simulink model "SAC_est_2d_test"  (R2025b)
settings: Solver=VariableStepAuto  StartTime=0.0  StopTime=300  FixedStep=1e-4  RelTol=1e-5
InitFcn:
  | % InitFcn (Model Properties > Callbacks > InitFcn)
  | 
  | % モデルファイルのフルパス（未保存だと空になるので注意）
  | % そのフォルダをパスに追加（重複追加はMATLAB側である程度防がれますが念のため）
  | modelDir = fileparts(get_param(bdroot, 'FileName'));
  | if ~contains(path, modelDir)
  |     addpath(modelDir);
  | end
  | 
  | % 呼びたい関数（そのフォルダ内に my_init.m がある想定）
  | model_init;  % 引数不要なら my_init; でもOK
model workspace (MAT data in the model file):
  ref_type = 1
values from neighbouring files (symbols this model uses):
  D = q(1)    [plantset.m]
  s = real2s(a, fmt) + real2s(b, fmt) + "i"    [plantset.m]
  Sm = zpk2struct([-0.7, -3]    , [-1.5, -7+3j, -7-3j], 1)    [plantset.m]
  Sp = Sp1    [plantset.m]
undefined symbols (not defined in the file or in its folder): a12, a22, Am, am, Am1, Am2, ampm, ap, Ap1, b1, b2, Bm, Bm1, Bm2, bp, Bp1, Cmdiag, DiscIntNeverNeededParam, dspblkCoreblockFVToolHelper, gcbh, ks, pdim, r_dim, rdim, sigamp, sigfreq, signormcoef, sigphs, Ts
libraries: simulink x13, ctrlSharedLib x1, slident x1, slctrl_signal x1, dspstat3 x1
settings Model: SimulationMode=accelerator  Creator=kawan  LastModifiedBy=kawan
settings SolverCC: ShapePreserveControl=EnableAll  ZeroCrossControl=DisableAll  ZeroCrossAlgorithm=Adaptive  MinimalZcImpactIntegration=on
settings DebuggingCC: ReadBeforeWriteMsg=DisableAll  WriteAfterWriteMsg=DisableAll  WriteAfterReadMsg=DisableAll  SolverPrmCheckMsg=warning  MultiTaskDSMMsg=none
settings ModelReferenceCC: UpdateModelReferenceTargets=IfOutOfDate
settings SFSimCC: SFSimEcho=off

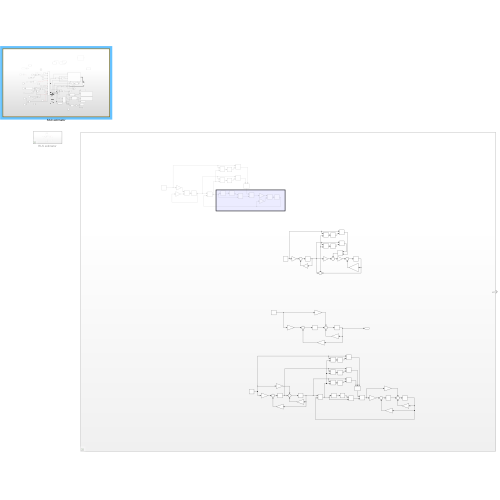
[thumbnail: Simulink's stored preview of the top-level diagram]
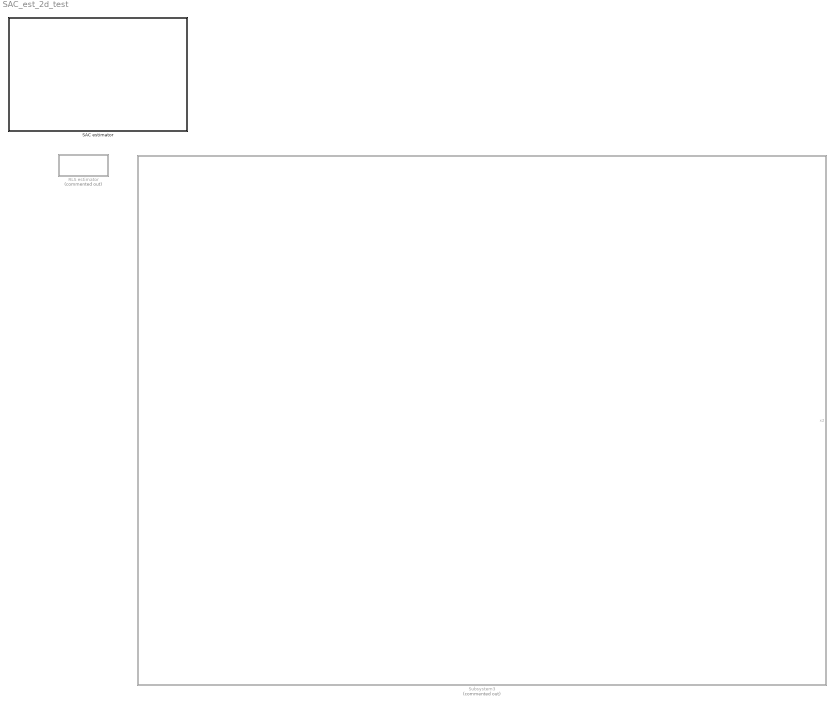
== system SAC_est_2d_test ==
  RLS estimator : Subsystem  Commented=on
  SAC estimator : Subsystem
  Subsystem3 : Subsystem  Commented=on

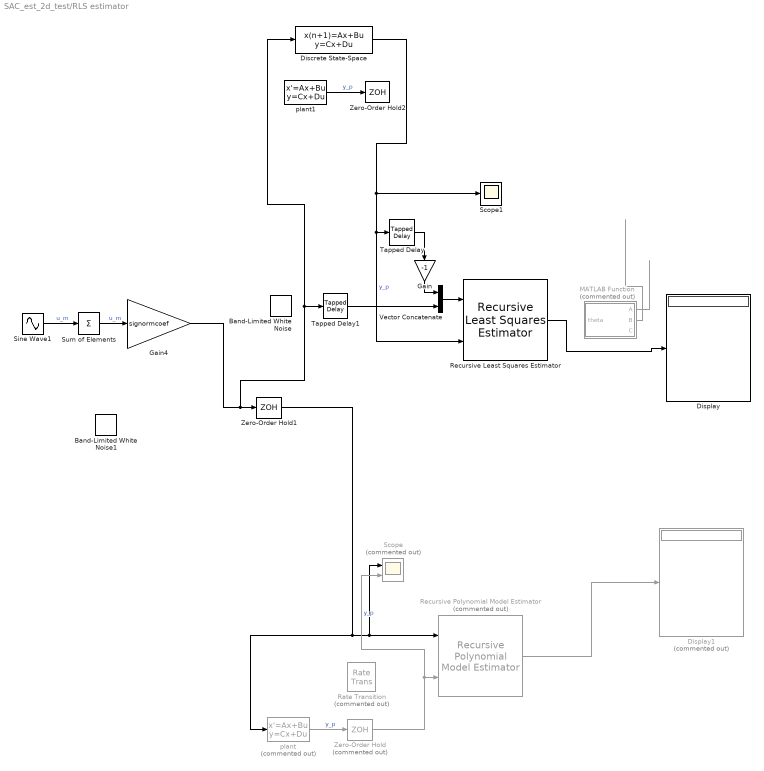
== system SAC_est_2d_test/RLS estimator ==
  Band-Limited White Noise : simulink/Sources/Band-Limited White Noise  Cov=[0.1]  Ts=Ts  seed=[23341]
  Band-Limited White Noise1 : simulink/Sources/Band-Limited White Noise  Cov=[0.1]  Ts=Ts  seed=[23341]
  Discrete State-Space : DiscreteStateSpace  A=[0 1 0; 0 0 1; -0.1 -0.5 -1.2]  B=[0; 0; 1]  C=[1.5 0.8 0]  D=0  SampleTime=Ts
  Display : Display
  Display1 : Display  Commented=on
  Gain : Gain  Gain=-1
  Gain4 : Gain  Gain=signormcoef
  MATLAB Function : MATLAB Function  Commented=on  TreatAsAtomicUnit=on
  Rate Transition : RateTransition  Commented=on  OutPortSampleTime=Ts
  Recursive Least Squares Estimator : ctrlSharedLib/Recursive Least Squares Estimator  InitialEstimateSource=Internal  InitialParameterData=[10000 10000 10000 10000 10000 10000]  P0=1e4  InitialRegressors=0  InitialOutputs=0  History=Infinite  WindowLength=200  EstimationMethod=Forgetting Factor  AdaptationParameter=lambda  HasTimeVaryingAdaptationParameter=off  NormalizationBias=eps  OutputError=off  OutputP=off  AddEnablePort=off  InputProcessing=Sample-based  Ts=-1
      settings: LibrarySourceBlock=slident/Estimators/Recursive Least Squares Estimator
  Recursive Polynomial Model Estimator : slident/Estimators/Recursive Polynomial Model Estimator  Commented=on  ModelStructure=ARX  InitialEstimateSource=None  A0=2  B0=2  C0=1  D0=1  F0=1  nk=1  P0=1e4  InitialInputs=0  InitialOutputs=0  History=Infinite  WindowLength=200  EstimationMethod=Forgetting Factor  AdaptationParameter=1  HasTimeVaryingAdaptationParameter=off  NormalizationBias=eps  OutputError=off  OutputP=off  AddEnablePort=off  InputProcessing=Sample-based  Ts=-1
  Scope : Scope  Commented=on  NumInputPorts=2
      settings: ActiveDisplayYMinimum=-1.1366422129559686  ActiveDisplayYMaximum=1.16288197779029  DataLoggingVariableName=ScopeData3
  Scope1 : Scope
      settings: DataLoggingVariableName=ScopeData5
  Sine Wave1 : Sin  Amplitude=sigamp  Frequency=sigfreq  Phase=sigphs  SampleTime=0
  Sum of Elements : Sum  Inputs=+
  Tapped Delay : simulink/Discrete/Tapped Delay  vinit=0.0  samptime=Ts  NumDelays=3  DelayOrder=Oldest  includeCurrent=off
  Tapped Delay1 : simulink/Discrete/Tapped Delay  vinit=0.0  samptime=Ts  NumDelays=3  DelayOrder=Oldest  includeCurrent=off
  Vector Concatenate : Concatenate
  Zero-Order Hold : ZeroOrderHold  Commented=on  SampleTime=Ts
  Zero-Order Hold1 : ZeroOrderHold  SampleTime=Ts
  Zero-Order Hold2 : ZeroOrderHold  SampleTime=Ts
  plant : StateSpace  Commented=on  A=Ap1  B=Bp1  C=[0 1]  D=0  InitialCondition=0
  plant1 : StateSpace  A=[0 1 0; 0 0 1; -0.1 -0.5 -1.2]  B=[0; 0; 1]  C=[1.5 0.8 0]  D=0  InitialCondition=0
  wires:
  Tapped Delay/1 -> Gain/1
  Gain4/1 -> Discrete State-Space/1, Tapped Delay1/1, Zero-Order Hold1/1
  Gain/1 -> Vector Concatenate/1
  Tapped Delay1/1 -> Vector Concatenate/2
  Vector Concatenate/1 -> Recursive Least Squares Estimator/1
  MATLAB Function/2(B) -> ?
  MATLAB Function/1(A) -> ?
  Recursive Least Squares Estimator/1 -> Display/1
  Sine Wave1/1 -> Sum of Elements/1  "u_m"
  Sum of Elements/1 -> Gain4/1  "u_m"
  Zero-Order Hold1/1 -> plant/1, Scope/1, Recursive Polynomial Model Estimator/1
  Recursive Polynomial Model Estimator/1 -> Display1/1
  Zero-Order Hold/1 -> Scope/2, Recursive Polynomial Model Estimator/2  "y_p"
  plant/1 -> Zero-Order Hold/1  "y_p"
  plant1/1 -> Zero-Order Hold2/1  "y_p"
  Discrete State-Space/1 -> Recursive Least Squares Estimator/2, Tapped Delay/1, Scope1/1  "y_p"

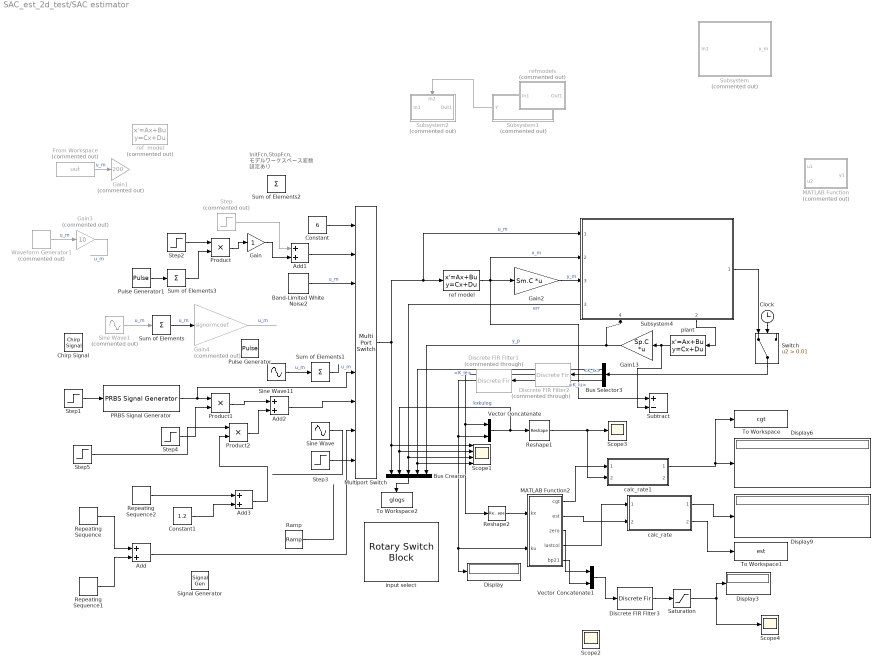
== system SAC_est_2d_test/SAC estimator ==
  note: InitFcn,StopFcn,
      | モデルワークスペース変数
      | 設定あり
  Add{,1..3} (4 alike) : Sum
  Band-Limited White Noise2 : simulink/Sources/Band-Limited White Noise  Cov=[0.1]  Ts=0.01  seed=[23490]
  Bus Creator : BusCreator  Inputs=5
  Bus Selector3 : BusSelector  OutputSignals=K_Ie,K_Ix,K_Iu
  Chirp Signal : simulink/Sources/Chirp Signal  f1=0.01  T=1000  f2=10
  Clock : Clock
  Constant : Constant  Value=6
  Constant1 : Constant  Value=1.2
  Discrete FIR Filter1 : DiscreteFir  Commented=through  LoadFcn=dspblkCoreblockFVToolHelper(gcbh,'load');  Coefficients=ones(1, 100)/100
      settings: CopyFcn=dspblkCoreblockFVToolHelper(gcbh,'copy');  DeleteFcn=dspblkCoreblockFVToolHelper(gcbh,'close');  ModelCloseFcn=dspblkCoreblockFVToolHelper(gcbh,'close');  PreSaveFcn=dspblkCoreblockFVToolHelper(gcbh,'presave');  PostSaveFcn=dspblkCoreblockFVToolHelper(gcbh,'postsave');  CloseFcn=dspblkCoreblockFVToolHelper(gcbh,'close');
  Discrete FIR Filter2 : DiscreteFir  Commented=through  LoadFcn=dspblkCoreblockFVToolHelper(gcbh,'load');  Coefficients=ones(1, 100)/100
      settings: CopyFcn=dspblkCoreblockFVToolHelper(gcbh,'copy');  DeleteFcn=dspblkCoreblockFVToolHelper(gcbh,'close');  ModelCloseFcn=dspblkCoreblockFVToolHelper(gcbh,'close');  PreSaveFcn=dspblkCoreblockFVToolHelper(gcbh,'presave');  PostSaveFcn=dspblkCoreblockFVToolHelper(gcbh,'postsave');  CloseFcn=dspblkCoreblockFVToolHelper(gcbh,'close');
  Discrete FIR Filter3 : DiscreteFir  LoadFcn=dspblkCoreblockFVToolHelper(gcbh,'load');  Coefficients=ones(1, 1000)/1000
      settings: CopyFcn=dspblkCoreblockFVToolHelper(gcbh,'copy');  DeleteFcn=dspblkCoreblockFVToolHelper(gcbh,'close');  ModelCloseFcn=dspblkCoreblockFVToolHelper(gcbh,'close');  PreSaveFcn=dspblkCoreblockFVToolHelper(gcbh,'presave');  PostSaveFcn=dspblkCoreblockFVToolHelper(gcbh,'postsave');  CloseFcn=dspblkCoreblockFVToolHelper(gcbh,'close');
  Display{,3,6,9} (4 alike) : Display
  From Workspace : FromWorkspace  Commented=on  VariableName=uut  SampleTime=0.01
  Gain : Gain
  Gain1 : Gain  Commented=on  Gain=200
  Gain13 : Gain  Gain=Sp.C  Multiplication=Matrix(K*u) (u vector)
  Gain2 : Gain  Gain=Sm.C  Multiplication=Matrix(K*u) (u vector)
  Gain3 : Gain  Commented=on  Gain=10
  Gain4 : Gain  Commented=on  Gain=signormcoef
  MATLAB Function : MATLAB Function  Commented=on  TreatAsAtomicUnit=on
  MATLAB Function2 : MATLAB Function  TreatAsAtomicUnit=on
  Multiport Switch : MultiPortSwitch  Inputs=8  SaturateOnIntegerOverflow=off  InputSameDT=off
  PRBS Signal Generator : slctrl_signal/PRBS Signal Generator  DiscreteTs=0.1  BlockDataType=double  SignalSource=Block parameters  Frequencies=[0.3 2 10 17 ]  FreqUnits=rad/s  Amplitudes=2  NumOfFreq=3  NumOfPRBSPeriod=2  UseAutogenNumOfPRBSPeriod=off  PRBSSignalOrder=12  UseAutogenPRBSSignalOrder=on  UseExternalTs=off  CompiledTsChoice=InternalTs
      settings: LibrarySourceBlock=slctrlblks/Signal Generation/PRBS Signal Generator
  Product : Product
  Product1 : Product
  Product2 : Product
  Pulse Generator : DiscretePulseGenerator  PulseType=Time based  Period=4  PulseWidth=50
  Pulse Generator1 : DiscretePulseGenerator  PulseType=Time based  Amplitude=[1 1 1 1 ]  Period=[3 7 11 29]  PulseWidth="[50 50 50  50]"  PhaseDelay=[0 0 0 0]
  Ramp : simulink/Sources/Ramp  slope=1  start=0  InitialOutput=0
  Repeating Sequence : simulink/Sources/Repeating Sequence  rep_seq_t=[0 1 2]  rep_seq_y=[-1 1 -1]
  Repeating Sequence1 : simulink/Sources/Repeating Sequence  rep_seq_t=[0 0.7 1.4]  rep_seq_y=[-1 1 -1]
  Repeating Sequence2 : simulink/Sources/Repeating Sequence  rep_seq_t=[0 40 80]  rep_seq_y=[-1 1 -1]
  Reshape1 : Reshape  OutputDimensionality=Column vector (2-D)
  Reshape2 : Reshape  OutputDimensionality=Row vector (2-D)
  Saturation : Saturate  UpperLimit=100  LowerLimit=-100
  Scope1 : Scope  NumInputPorts=4
      settings: ActiveDisplayYMinimum=-1.5374999999999999  ActiveDisplayYMaximum=3.8375000000000004  DataLoggingVariableName=ScopeData2
  Scope2 : Scope
      settings: ActiveDisplayYMinimum=-429.09941390661976  ActiveDisplayYMaximum=313.82518568676568
  Scope3 : Scope
      settings: ActiveDisplayYMinimum=-2.6867192013878816  ActiveDisplayYMaximum=2.9839772931263044  DataLoggingVariableName=ScopeData6
  Scope4 : Scope
      settings: ActiveDisplayYMinimum=-31.830161922792403  ActiveDisplayYMaximum=10.227460903276018  DataLoggingVariableName=ScopeData4
  Signal Generator : SignalGenerator  WaveForm=sawtooth  Amplitude=3  Units=rad/sec
  Sine Wave : Sin  Amplitude=2  Frequency=0.5  SampleTime=0
  Sine Wave1 : Sin  Commented=on  Amplitude=sigamp  Frequency=sigfreq  Phase=sigphs  SampleTime=0
  Sine Wave11 : Sin  Amplitude=[3 5 5 5 5]  Frequency=[3 1 0.6 0.08 0.05]  Phase=[0 0 1 2 3]  SampleTime=0
  Step : Step  Commented=on  Time=500  After=5  SampleTime=0
  Step1 : Step  SampleTime=0
  Step2 : Step  Time=100  Before=1  After=0  SampleTime=0
  Step3 : Step  After=15  SampleTime=0
  Step4 : Step  Time=100  Before=1  After=0  SampleTime=0
  Step5 : Step  Time=110  After=1.5  SampleTime=0
  Subsystem : Subsystem  Commented=on
  Subsystem1 : Subsystem  Commented=on
  Subsystem2 : Subsystem  Commented=on
      settings: PortSchema="{\"entries\":[{\"content\":{\"sides\":[{\"content\":{\"connectorIds\":[\"In1\"]},\"type\":\"ConnectorPlacement.EquallySpacedRectSide\",\"uuid\":\"ca1ca012-9e48-4d28-9546-9523a30e4c00\"},{\"content\":{\"connectorIds\":[\"Out1\"],\"side\":\"RIGHT\"},\"type\":\"ConnectorPlacement.EquallySpacedRectSide\",\"uuid\":\"6dfbe6e3-6ff1-4332-8540-578158e170be\"},{\"content\":{\"connectorIds\":[\"In2\"],\"side\":\"TOP\"},\"type\":\"ConnectorPlacement.EquallySpacedRectSide\",\"uuid\":\"173b116c-fc58-4287-8941-a18a90961935\"}]},\"type\":\"ConnectorPlacement.EquallySpacedConnector\",\"uuid\":\"dd7e7c07-a7d3-4b0a-ae00-63b25ccb3867\"}],\"packageUris\":[\"http://schema.mathworks.com/mf0/Connector/R2020b\"],\"version\":\"1.0\"}"
  Subsystem4 : Subsystem  ReferencedSubsystem=SAC_controller
      settings: PortSchema="{\"entries\":[{\"content\":{\"sides\":[{\"content\":{\"connectorIds\":[\"In1\",\"In2\",\"In3\",\"Out3\"]},\"type\":\"ConnectorPlacement.EquallySpacedRectSide\",\"uuid\":\"abf299e5-9df1-4fb5-aa74-01719925a1a1\"},{\"content\":{\"connectorIds\":[\"Out1\"],\"side\":\"RIGHT\"},\"type\":\"ConnectorPlacement.EquallySpacedRectSide\",\"uuid\":\"d214d5fa-0fee-4d3e-819e-59400150f2d9\"},{\"content\":{\"side\":\"TOP\"},\"type\":\"ConnectorPlacement.EquallySpacedRectSide\",\"uuid\":\"1eb393d4-8e3b-43af-9180-e24e7ecc06ed\"},{\"content\":{\"connectorIds\":[\"In4\",\"Out2\"],\"side\":\"BOTTOM\"},\"type\":\"ConnectorPlacement.EquallySpacedRectSide\",\"uuid\":\"f68492c4-4ddc-462c-84c1-db993ab53063\"}]},\"type\":\"ConnectorPlacement.EquallySpacedConnector\",\"uuid\":\"cd6940d7-fcf2-4cc0-908e-d3fd8a42eacf\"}],\"packageUris\":[\"http://schema.mathworks.com/mf0/Connector/R2020b\"],\"version\":\"1.0\"}"
  Subtract : Sum  Inputs=+-
  Sum of Elements{,1..3} (4 alike) : Sum  Inputs=+
  Switch : Switch  Criteria=u2 > Threshold  Threshold=0.01  SaturateOnIntegerOverflow=off  InputSameDT=off
  To Workspace : ToWorkspace  VariableName=cgt  SaveFormat=Structure With Time  SampleTime=-1
      settings: MaxDataPoints=1  Save2DSignal=2-D array (concatenate along first dimension)
  To Workspace1 : ToWorkspace  VariableName=est  SaveFormat=Structure With Time  SampleTime=-1
      settings: MaxDataPoints=1  Save2DSignal=2-D array (concatenate along first dimension)
  To Workspace2 : ToWorkspace  VariableName=glogs  SaveFormat=Timeseries  SampleTime=-1
      settings: Decimation=20
  Vector Concatenate : Concatenate
  Vector Concatenate1 : Concatenate
  Waveform Generator1 : simulink/Sources/Waveform Generator  Commented=on  OutMin=[]  OutMax=[]  OutDataTypeStr=double  SelectedSignal=1  Signals=sin(1,3,2)+sin(10, 10,0)+sin(5, 100,0)+ sin(5, 150, 1)  BlockNames=MultiportSwitch_32063c07ee454eb  SampleTime=0.001
  calc_rate : Subsystem  ReferencedSubsystem=calc_rate
  calc_rate1 : Subsystem  ReferencedSubsystem=calc_rate
  input select : RotarySwitchBlock
  plant : StateSpace  A=Sp.A  B=Sp.B  C=eye(rdim)  D=zeros(rdim,1)  InitialCondition=0
  ref  model : StateSpace  Commented=on  A=Am  B=Bm  C=Cmdiag  D=zeros(r_dim,1)  InitialCondition=0
  ref model : StateSpace  A=Sm.A  B=Sm.B  C=eye(pdim)  D=zeros(pdim,1)  InitialCondition=0
  refmodels : Subsystem  Commented=on  Variant=on  EmptyChoice=on
  wires:
  Add1/1 -> Multiport Switch/2
  ? -> Multiport Switch/4  "u_m"
  Sine Wave11/1 -> Sum of Elements1/1  "u_m"
  Switch/1 -> Bus Selector3/1
  Sine Wave1/1 -> Sum of Elements/1  "u_m"
  Gain3/1 -> ?  "u_m"
  Sum of Elements/1 -> Gain4/1  "u_m"
  MATLAB Function2/1(cgt) -> calc_rate1/1
  Constant/1 -> Multiport Switch/1
  Gain4/1 -> ?  "u_m"
  Subsystem4/1 -> Switch/1
  From Workspace/1 -> Gain1/1  "u_m"
  Sum of Elements1/1 -> ?  "u_m"
  Waveform Generator1/1 -> Gain3/1  "u_m"
  Sine Wave/1 -> ?
  Subsystem1/1(Y) -> Subsystem2/2(In2)
  Clock/1 -> Switch/2
  PRBS Signal Generator/1 -> Multiport Switch/6, Product1/1
  Step1/1 -> PRBS Signal Generator/1
  Multiport Switch/1 -> Subsystem4/1, ref model/1, Scope1/1, Bus Creator/1  "u_m"
  Step2/1 -> Product/1
  Step3/1 -> Multiport Switch/9
  Bus Selector3/2 -> Discrete FIR Filter2/1  "<K_Ix>"
  Bus Selector3/3 -> Discrete FIR Filter1/1  "<K_Iu>"
  Reshape2/1 -> MATLAB Function2/1(kx)
  ref model/1 -> Subsystem4/2, Subtract/1, Gain2/1  "x_m"
  Gain13/1 -> Bus Creator/5, Subsystem4/4  "y_p"
  plant/1 -> Subtract/2, Gain13/1
  Subsystem4/2 -> plant/1
  Gain2/1 -> Subsystem4/3  "y_m"
  Pulse Generator1/1 -> Sum of Elements3/1
  Sum of Elements3/1 -> Product/2
  Band-Limited White Noise2/1 -> Multiport Switch/3  "u_m"
  Vector Concatenate/1 -> Bus Creator/2, Scope1/2, Reshape1/1  "kxkulog"
  Subsystem4/3 -> Scope1/3, Bus Creator/3  "err"
  Product/1 -> Gain/1
  Bus Creator/1 -> To Workspace2/1
  Bus Selector3/1 -> Scope1/4, Bus Creator/4  "<K_Ie>"
  Step/1 -> Add1/1
  Saturation/1 -> Scope4/1, Display3/1
  Discrete FIR Filter2/1 -> Vector Concatenate/1, Reshape2/1
  Discrete FIR Filter1/1 -> Vector Concatenate/2, Display/1, MATLAB Function2/2(ku)
  calc_rate1/1 -> To Workspace/1, Display6/1
  Reshape1/1 -> calc_rate1/2, Scope3/1
  calc_rate/1 -> Display9/1
  MATLAB Function2/4(lastcol) -> calc_rate/1
  MATLAB Function2/2(est) -> calc_rate/2
  Gain/1 -> Add1/2
  calc_rate/2 -> To Workspace1/1
  Step4/1 -> Product1/2
  Step5/1 -> Product2/1
  Product1/1 -> Add2/1
  Add2/1 -> Multiport Switch/7
  MATLAB Function2/3(zero) -> Vector Concatenate1/1
  MATLAB Function2/5(bp21) -> Vector Concatenate1/2
  Vector Concatenate1/1 -> Discrete FIR Filter3/1
  Discrete FIR Filter3/1 -> Saturation/1
  Ramp/1 -> ?
  Add/1 -> Multiport Switch/8
  Repeating Sequence1/1 -> Add/2
  Repeating Sequence/1 -> Add/1
  Product2/1 -> Add2/2
  Repeating Sequence2/1 -> Add3/1
  Add3/1 -> Product2/2
  Constant1/1 -> Add3/2

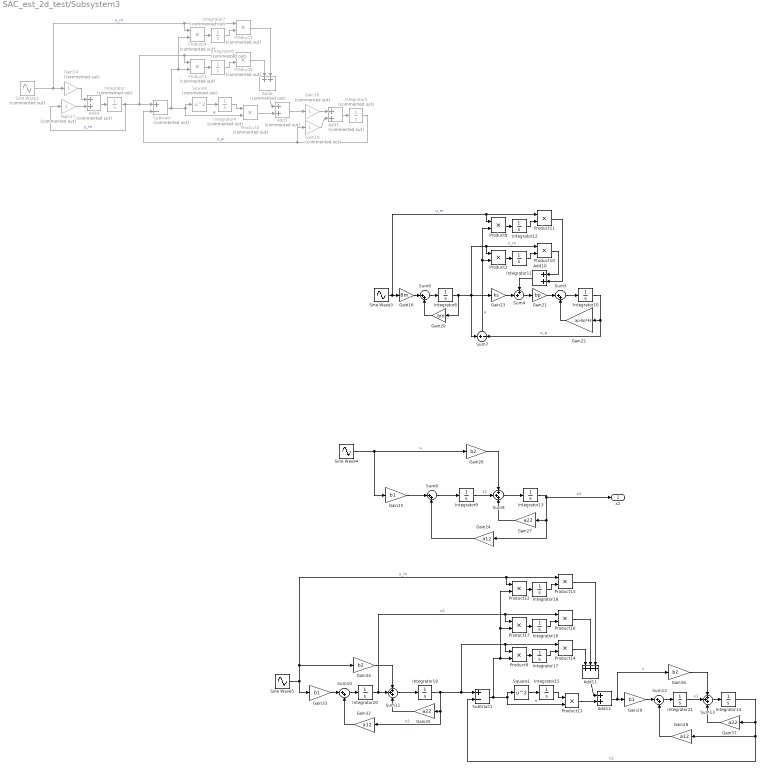
== system SAC_est_2d_test/Subsystem3 ==
  Add10 : Sum
  Add11 : Sum  Inputs=+++
  Add12 : Sum
  Add{4..7} (4 alike) : Sum  Commented=on
  Gain{14,17..19} (4 alike) : Gain  Commented=on
  Gain16 : Gain  Gain=Bm
  Gain20 : Gain  Gain=am
  Gain21 : Gain  Gain=bp
  Gain22 : Gain  Gain=ap-bp*ks
  Gain23 : Gain  Gain=ks
  Gain24 : Gain  Gain=a12
  Gain25 : Gain  Gain=b1
  Gain26 : Gain  Gain=b2
  Gain27 : Gain  Gain=a22
  Gain28 : Gain  Gain=a12
  Gain29 : Gain  Gain=b1
  Gain32 : Gain  Gain=a12
  Gain33 : Gain  Gain=b1
  Gain34 : Gain  Gain=b2
  Gain35 : Gain  Gain=a22
  Gain36 : Gain  Gain=b2
  Gain37 : Gain  Gain=a22
  Integrator{,4..7} (5 alike) : Integrator  Commented=on
  Integrator{8..21} (14 alike) : Integrator
  Product{2,8..17} (11 alike) : Product
  Product{3..7} (5 alike) : Product  Commented=on
  Sine Wave2 : Sin  Commented=on  SampleTime=0
  Sine Wave3 : Sin  SampleTime=0
  Sine Wave4 : Sin  SampleTime=0
  Sine Wave5 : Sin  SampleTime=0
  Square : Math  Commented=on  Operator=square
  Square1 : Math  Operator=square
  Subtract : Sum  Commented=on  Inputs=+-
  Subtract1 : Sum  Inputs=+-
  Sum{5..6,8,10,12} (5 alike) : Sum  Inputs=|++
  Sum11 : Sum  Inputs=+++
  Sum13 : Sum  Inputs=+++
  Sum4 : Sum  Inputs=++|
  Sum7 : Sum  Inputs=+|-
  Sum9 : Sum  Inputs=+++
  x2 : Outport
  wires:
  Sine Wave4/1 -> Gain26/1, Gain25/1  "u"
  Add4/1 -> Integrator/1
  Integrator12/1 -> Product11/2
  Subtract/1 -> Product5/2, Square/1, Product3/2, Product4/2  "e"
  Integrator/1 -> Gain17/1, Subtract/1, Product3/1, Product6/1  "y_m"
  Sum7/1 -> Product2/2, Product8/2  "e"
  Gain21/1 -> Sum5/1
  Integrator8/1 -> Sum7/1, Gain23/1, Product10/1, Product2/1, Gain20/1  "x_m"
  Sine Wave2/1 -> Gain14/1, Product7/1, Product4/1  "u_m"
  Add12/1 -> Gain29/1, Gain36/1  "u"
  Integrator20/1 -> Sum11/2, Product17/1, Product16/1  "x2"
  Integrator7/1 -> Product7/2
  Sine Wave3/1 -> Product11/1, Product8/1, Gain16/1  "u_m"
  Sine Wave5/1 -> Product15/1, Product12/1, Gain34/1, Gain33/1  "u_m"
  Integrator11/1 -> Product10/2
  Sum10/1 -> Integrator20/1
  Add10/1 -> Sum4/1
  Product7/1 -> Add6/2
  Sum6/1 -> Integrator8/1
  Gain24/1 -> Sum8/2
  Gain19/1 -> Add5/2
  Gain22/1 -> Sum5/2
  Product3/1 -> Integrator6/1
  Product8/1 -> Integrator12/1
  Integrator21/1 -> Sum13/2  "x1"
  Gain23/1 -> Sum4/2
  Square/1 -> Integrator4/1
  Sum4/1 -> Gain21/1
  Gain14/1 -> Add4/1
  Product11/1 -> Add10/2
  Integrator9/1 -> Sum9/2  "x1"
  Sum5/1 -> Integrator10/1
  Integrator4/1 -> Product5/1
  Integrator6/1 -> Product6/2
  Integrator5/1 -> Gain19/1, Subtract/2  "y_p"
  Add5/1 -> Integrator5/1
  Gain16/1 -> Sum6/1
  Product10/1 -> Add10/1
  Gain27/1 -> Sum9/3
  Integrator14/1 -> Subtract1/2, Gain28/1, Gain37/1  "x2"
  Integrator10/1 -> Sum7/2, Gain22/1  "x_p"
  Square1/1 -> Integrator15/1
  Gain33/1 -> Sum10/1
  Gain37/1 -> Sum13/3
  Integrator13/1 -> x2/1, Gain24/1, Gain27/1  "x2"
  Integrator18/1 -> Product15/2
  Sum9/1 -> Integrator13/1
  Gain20/1 -> Sum6/2
  Product6/1 -> Add6/1
  Gain18/1 -> Add5/1
  Product5/1 -> Add7/2
  Add7/1 -> Gain18/1
  Gain17/1 -> Add4/2
  Add6/1 -> Add7/1
  Product2/1 -> Integrator11/1
  Product9/1 -> Integrator17/1
  Product4/1 -> Integrator7/1
  Gain35/1 -> Sum11/3
  Sum8/1 -> Integrator9/1
  Gain32/1 -> Sum10/2
  Integrator19/1 -> Subtract1/1, Product9/1, Product14/1, Gain32/1, Gain35/1  "x2"
  Gain34/1 -> Sum11/1
  Sum11/1 -> Integrator19/1
  Subtract1/1 -> Product13/2, Square1/1, Product9/2, Product17/2, Product12/2  "e"
  Gain26/1 -> Sum9/1
  Gain25/1 -> Sum8/1
  Integrator17/1 -> Product14/2
  Integrator15/1 -> Product13/1
  Product16/1 -> Add11/2
  Gain29/1 -> Sum12/1
  Product13/1 -> Add12/2
  Product12/1 -> Integrator18/1
  Add11/1 -> Add12/1
  Product15/1 -> Add11/3
  Product14/1 -> Add11/1
  Integrator16/1 -> Product16/2
  Product17/1 -> Integrator16/1
  Gain28/1 -> Sum12/2
  Gain36/1 -> Sum13/1
  Sum13/1 -> Integrator14/1
  Sum12/1 -> Integrator21/1

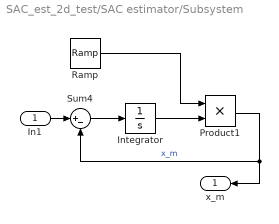
== system SAC_est_2d_test/SAC estimator/Subsystem ==
  In1 : Inport
  Integrator : Integrator
  Product1 : Product
  Ramp : simulink/Sources/Ramp  slope=-0.01  start=0  InitialOutput=-40
  Sum4 : Sum  Inputs=|+-
  x_m : Outport
  wires:
  Integrator/1 -> Product1/2
  Sum4/1 -> Integrator/1
  Product1/1 -> x_m/1, Sum4/2  "x_m"
  In1/1 -> Sum4/1
  Ramp/1 -> Product1/1

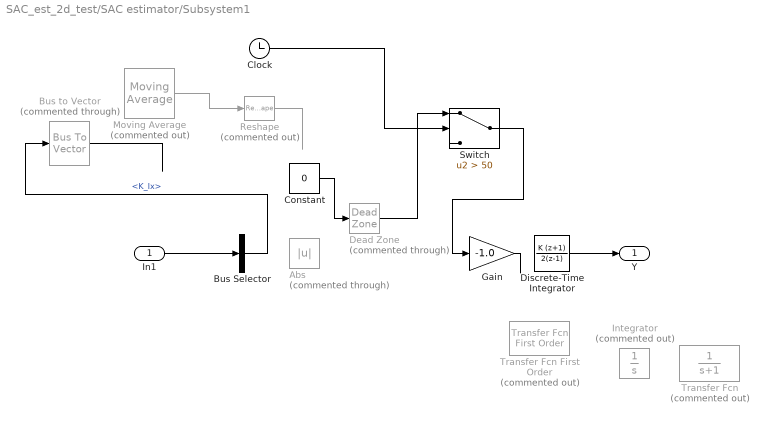
== system SAC_est_2d_test/SAC estimator/Subsystem1 ==
  In1 : Inport
  Abs : Abs  Commented=through  SaturateOnIntegerOverflow=off
  Bus Selector : BusSelector  OutputSignals=K_Ix
  Bus to Vector : BusToVector  Commented=through
  Clock : Clock
  Constant : Constant  Value=0
  Dead Zone : DeadZone  Commented=through  LowerValue=-0.00001  UpperValue=0.00001
  Discrete-Time Integrator : DiscreteIntegrator  IntegratorMethod=Accumulation: Trapezoidal  InitialCondition=ampm  SampleTime=-1  ICPrevOutput=DiscIntNeverNeededParam  ICPrevScaledInput=DiscIntNeverNeededParam
  Gain : Gain  Gain=-1.0
  Integrator : Integrator  Commented=on  InitialCondition=[-30.0 -55.0 -80.0]
  Moving Average : dspstat3/Moving Average  Commented=on  Method=Sliding window  ForgettingFactorPort=off  SpecifyWindowLength=on  WindowLength=501  OverlapLength=500  AllowArbitraryInputLength=off  ForgettingFactor=0.9  SimulateUsing=Code generation
  Reshape : Reshape  Commented=on
  Switch : Switch  Criteria=u2 > Threshold  Threshold=50  SaturateOnIntegerOverflow=off  InputSameDT=off
  Transfer Fcn : TransferFcn  Commented=on  Denominator=[1 1]
  Transfer Fcn First Order : simulink/Discrete/Transfer Fcn First Order  Commented=on  PoleZ=0.95  ICPrevOutput=[-30.0 -55.0 -80.0]  DoSatur=off
  Y : Outport
  wires:
  In1/1 -> Bus Selector/1
  Gain/1 -> ?
  Bus Selector/1 -> Bus to Vector/1  "<K_Ix>"
  Constant/1 -> Dead Zone/1
  Discrete-Time Integrator/1 -> Y/1
  Dead Zone/1 -> Switch/1
  Bus to Vector/1 -> ?
  Moving Average/1 -> Reshape/1
  Clock/1 -> Switch/2
  Switch/1 -> Gain/1
  Reshape/1 -> ?

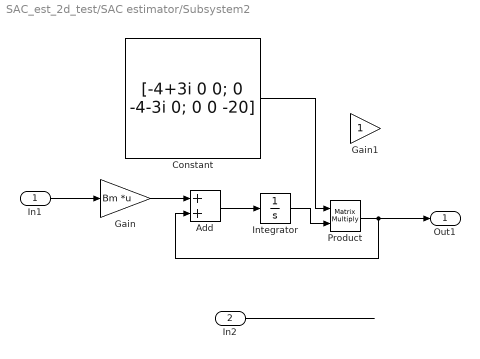
== system SAC_est_2d_test/SAC estimator/Subsystem2 ==
  In1 : Inport
  In2 : Inport  Port=2
  Add : Sum
  Constant : Constant  Value=[-4+3i 0 0; 0 -4-3i 0; 0 0 -20]
  Gain : Gain  Gain=Bm  Multiplication=Matrix(K*u)
  Gain1 : Gain
  Integrator : Integrator
  Product : Product  Multiplication=Matrix(*)
  Out1 : Outport
  wires:
  In2/1 -> ?
  Integrator/1 -> Product/2
  Gain/1 -> Add/1
  Product/1 -> Add/2, Out1/1
  Add/1 -> Integrator/1
  In1/1 -> Gain/1
  Constant/1 -> Product/1

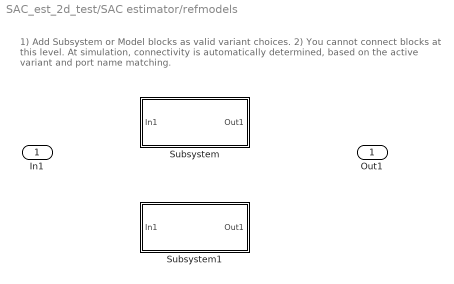
== system SAC_est_2d_test/SAC estimator/refmodels ==
  note: 1) Add Subsystem or Model blocks as valid variant choices.
      | 2) You cannot connect blocks at this level. At simulation, connectivity is automatically
      | determined, based on the active variant and port name matching.
  In1 : Inport
  Subsystem : Subsystem  VariantControl=ref_type == 1
  Subsystem1 : Subsystem  VariantControl=ref_type == 2
  Out1 : Outport

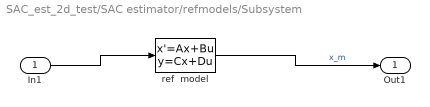
== system SAC_est_2d_test/SAC estimator/refmodels/Subsystem ==
  In1 : Inport
  ref  model : StateSpace  A=Am1  B=Bm1  C=Cmdiag  D=zeros(r_dim,1)  InitialCondition=0
  Out1 : Outport
  wires:
  In1/1 -> ref  model/1
  ref  model/1 -> Out1/1  "x_m"

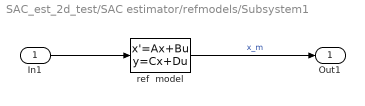
== system SAC_est_2d_test/SAC estimator/refmodels/Subsystem1 ==
  In1 : Inport
  ref  model : StateSpace  A=Am2  B=Bm2  C=Cmdiag  D=zeros(r_dim,1)  InitialCondition=0
  Out1 : Outport
  wires:
  In1/1 -> ref  model/1
  ref  model/1 -> Out1/1  "x_m"

== matlab function SAC_est_2d_test/RLS estimator/MATLAB Function ==
  data: theta input; A output; B output; C output
function [A, B, C] = arx2ss(theta)
    % theta = [a1, a2, a3, b1, b2, b3]
    % ※入力順序はVector Concatenateの接続順に依存します。
    %   ここでは前半3つがa、後半3つがbと想定しています。

    a1 = theta(1);
    a2 = theta(2);
    %a3 = theta(3);
    b1 = theta(4);
    b2 = theta(5);
    %b3 = theta(6);

    % 可観測正準形
    A = [ -a1   1   0;
          -a2   0   1;
          -a3   0   0 ];
          
    B = [ b1;
          b2;
          b3 ];
          
    C = [ 1   0   0 ];
    
    % D行列が必要な場合は別途推定が必要ですが、今回はD=0と仮定
end

== matlab function SAC_est_2d_test/SAC estimator/MATLAB Function ==
  data: u1 input; y1 output; u2 input
function y1 = fcn(u1, u2)

y1 = 0.5*sqrt(u1^2 + u2^2);

== matlab function SAC_est_2d_test/SAC estimator/MATLAB Function2 ==
  data: cgt output; est output; kx input; ku input; zero output; lastcol output; Sp parameter; Sm parameter; bp21 output
function [cgt, est, zero, lastcol, bp21]= fcn(kx, ku, Sp, Sm)

cgt_expr = @(am,bm,ap,bp) [am(1,2).*bp(2,1) - am(2,2).*bp(1,1) bp(1,1) 0; bp(1,1) bp(2,1) 0; bm(1,1).*bp(2,1) - bm(2,1).*bp(1,1) 0 bp(1,1)] \ [am(1,2) - ap(1,2); am(2,2) - ap(2,2); bm(1,1)];
est_expr = @(am,bm,bp,kx,ku) -1*[-am(2,2).*kx(1,1) + kx(1,2) am(1,2).*kx(1,1); kx(1,1) kx(1,2); -bm(2,1).*kx(1,1) + ku(1,1) bm(1,1).*kx(1,1)]*[bp(1,1); bp(2,1)] + [am(1,2); am(2,2); bm(1,1)];

cgt     = cgt_expr(Sm.A, Sm.B, Sp.A, Sp.B);
esttemp = est_expr(Sm.A, Sm.B, (Sm.B)./ku, kx, ku);

est = esttemp(1:end-1, :);
zero = esttemp(end, :)*1e5;
lastcol = Sp.A(:, end);

bp11 = Sm.B(1,1) / ku(1,1);

a = -1*Sm.B(2,1)*kx(1,1)+ku(1,1);
b = Sm.B(1,1)*kx(1,1);

bp21 = (Sm.B(1,1) - a*bp11) / (b);
